simulink model "Res_23"  (R2018b)
settings: Solver=ode4  StartTime=0.0  StopTime=1.5  FixedStep=2e-4  RelTol=1e-3  EnableMultiTasking=on
values from neighbouring files (symbols this model uses):
  A = [ 0 1 0 0 ; -k1/m1 -b/m1 k1/m1 b/m1 ; 0 0 0 1 ; k1/m2 b/m2 (-k1-k2)/m2 -b/m2 ]    [result_23.m]
  B = [ 0 ; 0 ; 0 ; k2/m2 ]    [result_23.m]
  C = [ 1 0 -1 0 ; 0 1 0 -1 ]    [result_23.m]
  D = [ 0 ; 0 ]    [result_23.m]
settings Model: Creator=makha  LastModifiedBy=makha

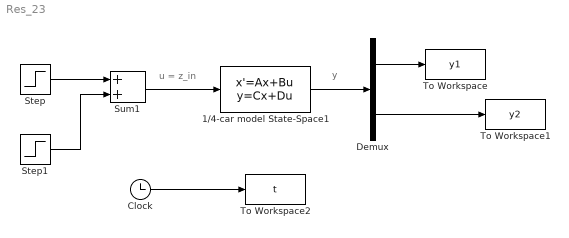
== system Res_23 ==
  note: y
  note: u = z_in
  1/4-car model State-Space1 : StateSpace  A=A  B=B  C=C  D=D  InitialCondition=zeros(4,1)
  Clock : Clock
  Demux : Demux  Outputs=2
  Step : Step  Time=0  After=0.1  SampleTime=0
  Step1 : Step  Time=0.01491  After=-0.1  SampleTime=0
  Sum1 : Sum
  To Workspace : ToWorkspace  VariableName=y1  SampleTime=-1
  To Workspace1 : ToWorkspace  VariableName=y2  SampleTime=-1
  To Workspace2 : ToWorkspace  VariableName=t  SampleTime=-1
  wires:
  Demux/1 -> To Workspace/1
  Step1/1 -> Sum1/2
  Step/1 -> Sum1/1
  Clock/1 -> To Workspace2/1
  Demux/2 -> To Workspace1/1
  Sum1/1 -> 1/4-car model State-Space1/1
  1/4-car model State-Space1/1 -> Demux/1
